simulink model "OFDM"  (R2020b)
settings: Solver=VariableStepDiscrete  StartTime=0.0  StopTime=inf  RelTol=1e-3
PreLoadFcn:
  | N = 64;
  | TsOFDM = 3.2e-6;
  | nb_pilotes = 16;
  | sample_time = TsOFDM/(2*N);
  | nb_pc = 4;
InitFcn:
  | N = 64;
  | TsOFDM = 3.2e-6;
  | nb_pilotes = 16;
  | sample_time = TsOFDM/(2*N);
  | nb_pc = 4;
undefined symbols (not defined in the file or in its folder): doppler
libraries: dspindex x4, dspxfrm3 x2, commdigbbndpm3 x2, commrandsrc3 x1, commsink2 x1, commchan3 x1
settings Model: Creator=t_issarni  LastModifiedBy=ncavalier
settings DataIOCC: LimitDataPoints=on  SaveOutput=off  SaveTime=off
settings OptimizationCC: BooleanDataType=off  DefaultParameterBehavior=Inlined  LocalBlockOutputs=off  LifeSpan=inf
settings DebuggingCC: AlgebraicLoopMsg=error  SingleTaskRateTransMsg=error  AllowSymbolicDim=off  SFUnexpectedBacktrackingDiag=warning  SFNoUnconditionalDefaultTransitionDiag=warning  SFExecutionAtInitializationDiag=none  ArithmeticOperatorsInVariantConditions=warning
settings SFSimCC: SimUseLocalCustomCode=off  CustomCodeUndefinedFunction=UseInterfaceOnly
settings RTWCC: RTWUseLocalCustomCode=off
settings CodeAppCC: StateflowObjectComments=on
settings GRTTargetCC: TargetLangStandard=C89/C90 (ANSI)
settings ConfigComp: CovMetricSettings=dw  CovSaveCumulativeToWorkspaceVar=on  CovSaveSingleToWorkspaceVar=on  CovExternalEMLEnable=off  CovSFcnEnable=off

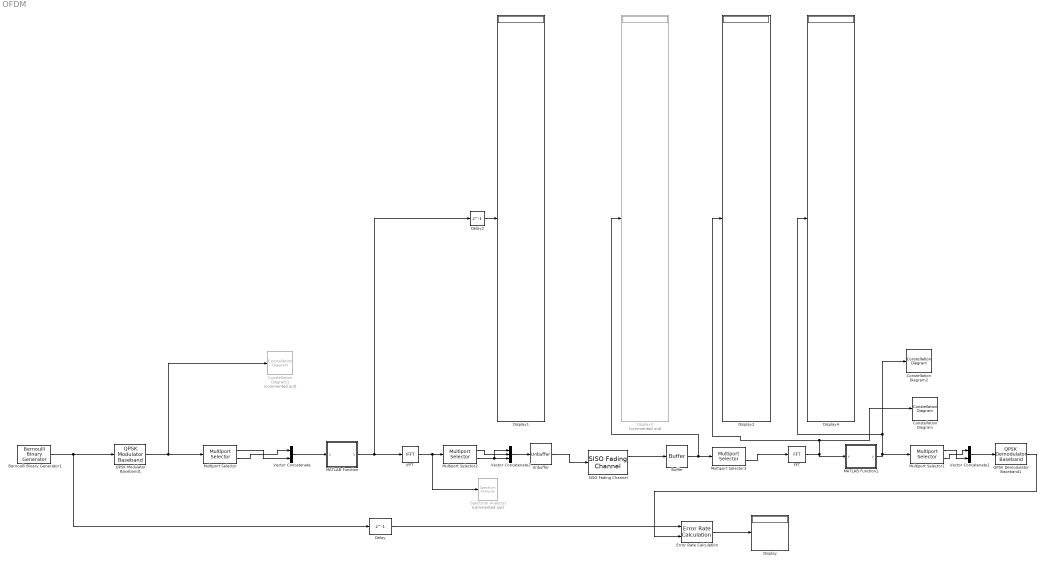
== system OFDM ==
  Bernoulli Binary Generator1 : commrandsrc3/Bernoulli Binary Generator  ProbabilityOfZero=0.5  SeedSource=Parameter  Seed=randi(100)  SampleTime=TsOFDM/(2*(N-nb_pilotes-nb_pc))  SamplesPerFrame=2*(N - nb_pilotes-nb_pc)  OutputDataType=double  SimulateUsing=Code generation
  Buffer : Buffer  OutputFrames=off
  Constellation Diagram : ConstellationDiagram
  Constellation Diagram1 : ConstellationDiagram  Commented=on
  Constellation Diagram2 : ConstellationDiagram
  Delay : Delay  DelayLength=1  InitialCondition=0  UseCircularBuffer=on
  Delay2 : Delay  DelayLength=1
  Display{,1..2,4} (4 alike) : Display
  Display3 : Display  Commented=on
  Error Rate Calculation : commsink2/Error Rate Calculation  N=0  st_delay=0  cp_mode=Entire frame  subframe=[]  PMode=Port  WsName=ErrorVec  RsMode2=off  stop=off  numErr=100  maxBits=1e6
      settings: SourceProductName=Communications Toolbox
  FFT : dspxfrm3/FFT  FFTImplementation=Auto  CompMethod=Table lookup  TableOpt=NEW  TableOptActive=Speed  BitRevOrder=off  Normalize=off  InheritFFTLength=on  FFTLength=64  WrapInput=on  roundingMode=Floor  overflowMode=off  firstCoeffDataTypeStr=Inherit: Same word length as input  firstCoeffLastDataTypeStr=Inherit: Same word length as input  outputMin=[]  outputMax=[]
  IFFT : dspxfrm3/IFFT  FFTImplementation=Auto  CompMethod=Table lookup  TableOpt=NEW  TableOptActive=Speed  BitRevOrder=off  cs_in=off  Normalize=on  InheritFFTLength=on  FFTLength=64  WrapInput=on  mode=Complex  outSamplingMode=Sample based  roundingMode=Floor  overflowMode=off  firstCoeffDataTypeStr=Inherit: Same word length as input  firstCoeffLastDataTypeStr=Inherit: Same word length as input  outputMin=[]  outputMax=[]
  MATLAB Function : MATLAB Function  TreatAsAtomicUnit=on
  MATLAB Function1 : MATLAB Function  TreatAsAtomicUnit=on
  Multiport Selector : dspindex/Multiport Selector  rowsOrCols=Rows  idxCellArray="{1 : (N-nb_pilotes-nb_pc)/2,  ((N-nb_pilotes-nb_pc)/2) + 1 : N-nb_pilotes-nb_pc}"  idxErrMode=Clip Index
  Multiport Selector1 : dspindex/Multiport Selector  rowsOrCols=Rows  idxCellArray="{1 : (N-nb_pilotes-nb_pc)/2,  ((N-nb_pilotes-nb_pc)/2) + 1 : N-nb_pilotes-nb_pc}"  idxErrMode=Clip Index
  Multiport Selector2 : dspindex/Multiport Selector  rowsOrCols=Rows  idxCellArray="{1 : (N - 2*nb_pc),  ((N-2*nb_pc)) + 1 : N-nb_pc}"  idxErrMode=Clip Index
  Multiport Selector3 : dspindex/Multiport Selector  rowsOrCols=Rows  idxCellArray="{1 : (nb_pc),  nb_pc + 1 : N}"  idxErrMode=Clip Index
  QPSK Demodulator Baseband1 : commdigbbndpm3/QPSK Demodulator Baseband  OutType=Bit  DecType=Hard decision  VarSource=Dialog  Variance=1  Dec=Gray  Ph=pi/4  outDtype1=Inherit via internal rule  outDtype2=Inherit via internal rule  derotateFactorWordLen=16  derotateFactorDataTypeStr=Inherit: Same word length as input  derotateFactorLastDataTypeStr=Inherit: Same word length as input
      settings: SourceProductName=Communications Toolbox
  QPSK Modulator Baseband1 : commdigbbndpm3/QPSK Modulator Baseband  InType=Bit  Enc=Gray  Ph=pi/4  outDtype=double  outWordLen=16  outUDDataType=sfix(16)  outFracLenMode=Best precision  outFracLen=15  outDataTypeStr=double  outLastDataTypeStr=double
      settings: SourceProductName=Communications Toolbox
  SISO Fading Channel : commchan3/SISO Fading Channel  InheritSampleRate=on  SampleRate=1  PathDelays=[0 4*(TsOFDM/N)]  AveragePathGains=[0 -3]  NormalizePathGains=on  FadingDistribution=Rayleigh  KFactor=3  DirectPathDopplerShift=0  DirectPathInitialPhase=0  MaximumDopplerShift=100  DopplerSpectrum=doppler('Jakes')  RandomStream=mt19937ar with seed  Seed=randi(1000)  PathGainsOutputPort=on  ChannelFilterDelayOutputPort=off  SimulateUsing=Code generation  Visualization=Off  PathsForDopplerDisplay=1  SamplesToDisplay=25%
  Spectrum Analyzer : SpectrumAnalyzer  Commented=on
  Unbuffer : Unbuffer
  Vector Concatenate : Concatenate
  Vector Concatenate1 : Concatenate
  Vector Concatenate2 : Concatenate  NumInputs=3
  wires:
  Bernoulli Binary Generator1/1 -> QPSK Modulator Baseband1/1, Delay/1
  Vector Concatenate/1 -> MATLAB Function/1(u)
  MATLAB Function1/1(y) -> Multiport Selector1/1, Display4/1, Constellation Diagram2/1
  MATLAB Function/1(y) -> IFFT/1, Delay2/1
  QPSK Modulator Baseband1/1 -> Multiport Selector/1, Constellation Diagram1/1
  Multiport Selector/2 -> Vector Concatenate/1
  Delay2/1 -> Display1/1
  Vector Concatenate1/1 -> QPSK Demodulator Baseband1/1
  Multiport Selector/1 -> Vector Concatenate/2
  Multiport Selector1/2 -> Vector Concatenate1/1
  Multiport Selector1/1 -> Vector Concatenate1/2
  FFT/1 -> Display2/1, Constellation Diagram/1, MATLAB Function1/1(x)
  Error Rate Calculation/1 -> Display/1
  Unbuffer/1 -> SISO Fading Channel/1
  Buffer/1 -> Multiport Selector3/1, Display3/1
  SISO Fading Channel/1 -> Buffer/1
  IFFT/1 -> Multiport Selector2/1, Spectrum Analyzer/1
  Vector Concatenate2/1 -> Unbuffer/1
  Multiport Selector3/2 -> FFT/1
  Multiport Selector2/2 -> Vector Concatenate2/3, Vector Concatenate2/1
  Multiport Selector2/1 -> Vector Concatenate2/2
  Delay/1 -> Error Rate Calculation/1
  QPSK Demodulator Baseband1/1 -> Error Rate Calculation/2

== matlab function OFDM/MATLAB Function1 ==
  data: x input; y output; nb_pilotes parameter; N parameter; nb_pc parameter
function y = fcn(x, nb_pilotes, N, nb_pc)
y = complex(zeros(N-nb_pilotes-nb_pc,1));
samples_out = complex(zeros(N-nb_pilotes-nb_pc,1));
samples = complex(zeros(N-nb_pilotes-nb_pc,1));
pilotes = complex(zeros(nb_pilotes,1));
pas = ceil((N-nb_pc)/nb_pilotes);


last_idx_pilote = 1;
last_idx_sample = 1; 
% on sépare les pilotes et les échantillons
for i=1:N-nb_pc
    if mod(i-1,pas) == 0 || last_idx_sample > N-nb_pilotes-nb_pc
        pilotes(last_idx_pilote, 1) = x(i,1);
        last_idx_pilote = last_idx_pilote +1;

    else      
        samples(last_idx_sample, 1) = complex(x(i,1));
        last_idx_sample = last_idx_sample +1;
    end
end


nb_samples_parcouru = 0;
pilotes_parcouru = 0;
for i=1:nb_pilotes - 1
    ecart = pas;
    if nb_samples_parcouru >= N-nb_pilotes-nb_pc - (pas-1)
        ecart = N-nb_pilotes-nb_pc - nb_samples_parcouru + 1;
    end
    
    pente_RE = (real(pilotes(pilotes_parcouru + 2, 1)) - real(pilotes(pilotes_parcouru + 1, 1))) / ecart;
    pente_IM = (imag(pilotes(pilotes_parcouru + 2, 1)) - imag(pilotes(pilotes_parcouru + 1, 1))) / ecart;
    x = 0:ecart;
    equation_pente_real = pente_RE*x + real(pilotes(pilotes_parcouru + 1, 1));
    equation_pente_imag = pente_IM*x + imag(pilotes(pilotes_parcouru + 1, 1));
    coef_interpo = complex(zeros(ecart+1,1));
    
    % calcul coefficients d'interpollation
    for p=1:ecart+1
        coef_interpo(p,1) = complex(equation_pente_real(1,p), equation_pente_imag(1,p));
    end
    

    for j=1:pas-1
        % calcul interpollation
        if nb_samples_parcouru < N-nb_pilotes-nb_pc
            samples_out((i-1)*(pas-1) + j,1) = samples((i-1)*(pas-1) + j,1) / coef_interpo(j+1,1);
            nb_samples_parcouru = nb_samples_parcouru + 1;
        end
    
    end
    
    pilotes_parcouru = pilotes_parcouru + 1;
end




% 
% % on calcule la phase et le module de chaque échantillon
% for i=1:N-nb_pilotes-nb_pc
%     modules(i,1) = abs(samples_out(i,1));
%     phases(i,1) = angle(samples_out(i,1));
% end


% compteur = 1;
% pilotes_parcouru = 0;
% nb_samples_parcouru = 0;
% for i=1:nb_pilotes - 1
%     
% %     if pilotes_parcouru < nb_pilotes - 1 
%         ecart = pas;
%         if nb_samples_parcouru >= N-nb_pilotes-nb_pc - (pas-1)
%             ecart = N-nb_pilotes-nb_pc - nb_samples_parcouru + 1;
%         end
%         
%         pente_module = (abs(pilotes(pilotes_parcouru + 2, 1)) - abs(pilotes(pilotes_parcouru + 1, 1))) / ecart;
%         pente_phase = (angle(pilotes(pilotes_parcouru + 2, 1)) - angle(pilotes(pilotes_parcouru + 1, 1))) / ecart;
%         
%         x = 0:ecart;
%         equation_pente_module = pente_module*x + abs(pilotes(pilotes_parcouru + 1, 1));
%         equation_pente_phase = pente_phase*x + angle(pilotes(pilotes_parcouru + 1, 1));
%         
%         
%         for j=1:pas-1
%             % calcul sur chaque coeff
%             if nb_samples_parcouru < N-nb_pilotes-nb_pc
%                 coef_IL_mod(compteur,1) = modules((pilotes_parcouru * (pas-1)) + j,1) / equation_pente_module(1,j+1);
%                 coef_IL_phase(compteur,1) = phases((pilotes_parcouru * (pas-1)) + j,1) - equation_pente_phase(1,j+1);
%                 nb_samples_parcouru = nb_samples_parcouru + 1;
%             end
%             
%             compteur = compteur + 1;
%         end
%         
%         pilotes_parcouru = pilotes_parcouru + 1;
%         
%         
% %     else
% %         % pente constante
% %         pente_module = abs(pilotes(pilotes_parcouru, 1));
% %         pente_phase = angle(pilotes(pilotes_parcouru, 1));
% %         for j=1:pas-1
% %             % calcul sur chaque coeff
% %             disp('____________-')
% %             coef_IL_mod(compteur,1) = modules((pilotes_parcouru * (pas-1)) + j,1) / pente_module;
% %             disp(coef_IL_mod(compteur,1))
% %             coef_IL_phase(compteur,1) = phases((pilotes_parcouru * (pas-1)) + j,1) - pente_phase;
% %             disp(coef_IL_phase(compteur,1))
% %             compteur = compteur + 1;
% %         end
% %         
% %     end
%  
% end
% 
% 
% % on assemble partie réelle et imaginaire
% for j=1:N-nb_pilotes-nb_pc
%     
%     if (modules(j,1) && phases(j,1)) ~= 0
%         samples_out(j,1) = coef_IL_mod(j,1)*(cos(coef_IL_phase(j,1)) + complex(0,1)* sin(coef_IL_phase(j,1)));
%     else
%         samples_out(j,1) = 0;
%     end
%     
% end
% 
% 
% %
% % compteur_tour = 1;
% % for i=1:nb_pilotes
% %     for j=1:pas
% %         if i == nb_pilotes 
% %             if compteur_tour > size(coef_IL_mod)
% %                break
% %             else 
% %                 disp("hello");
% %                 coef_IL_mod(compteur_tour, 1) = modules(i,1);
% %                 coef_IL_phase(compteur_tour, 1) = phases(i,1);
% %                 disp(coef_IL_mod(compteur_tour, 1));
% %                 compteur_tour = compteur_tour + 1;
% %             end
% %         else 
% %             disp(compteur_tour);
% %             coef_IL_mod(compteur_tour, 1) = modules(i,1) + ((modules(i+1,1)-modules(i,1))/(pas-2))*(j-1);
% %             coef_IL_phase(compteur_tour, 1) = phases(i,1) + ((phases(i+1,1)-phases(i,1))/(pas-2))*(j-1);
% % 
% %             disp((modules(i+1,1)-modules(i,1))/(pas-1));
% %             compteur_tour = compteur_tour + 1;
% %         end 
% %     end
% % end
% % 
% % 
% % for i=1:compteur_tour-1
% %     disp(coef_IL_mod(i,1));
% %     samples_out(i, 1) = (samples_out(i, 1) / coef_IL_mod(i, 1));
% % end
% % 
% 
% %4*(TsOFDM/N)

y = samples_out;

== matlab function OFDM/MATLAB Function ==
  data: u input; y output; nb_pilotes parameter; N parameter; nb_pc parameter
function y = fcn(u, nb_pilotes, N, nb_pc)

samples_in = complex(u);
samples_out = complex(zeros(N-nb_pc,1));


pas = ceil((N-nb_pc)/nb_pilotes);
last_idx = 1;
for i=1:N - nb_pc
 
    if (mod(i-1,pas) == 0) || (last_idx > N-nb_pilotes-nb_pc)
        samples_out(i,1) = complex(1,i*0);
    else
        samples_out(i,1) = samples_in(last_idx,1);
        last_idx = last_idx + 1;
    end
   
end



y = samples_out;
